simulink model "model_sim_CHBjt9"  (R2023b)
settings: Solver=FixedStepAuto  StartTime=0.0  StopTime=5  FixedStep=1e-6  RelTol=1e-3
InitFcn:
  | sysinit
values from neighbouring files (symbols this model uses):
  C = 0.0234    [sysinit.m]
  f_m = frequency_modulate_start : frequency_modulate_interval : frequency_modulate_end    [simout_chbjt_par.m]    (also in simresjt7.mat = [250 300 350 400 450 500 550 600 650 700 750 800 ... (16 ele)
  L = 0.002    [sysinit.m]
  m = modulate_radio_start : modulate_radio_interval : modulate_radio_end    [simout_chb_par.m]
  R = 1.5    [sysinit.m]
  st = 1e-6    (= 1e-06)    [sysinit.m]
undefined symbols (not defined in the file or in its folder): f, magnitude, Td, Ts2, udc
libraries: spsSeriesRLCBranchLib x123, spsDiodeLib x60, spsIGBTLib x48, spsMeanLib x20, spsCurrentMeasurementLib x16, spsThreePhaseVIMeasurementLib x13, spsOnDelayLib x12, spsUniversalBridgeLib x12, spsMultiWindingTransformerLib x9, spsVoltageMeasurementLib x6, simulink x5, spsPowerLib x2
(part 1 of 3)
settings Model: Creator=Jhchen  LastModifiedBy=ps
settings DataIOCC: ReturnWorkspaceOutputs=off
settings DebuggingCC: RTPrefix=warning

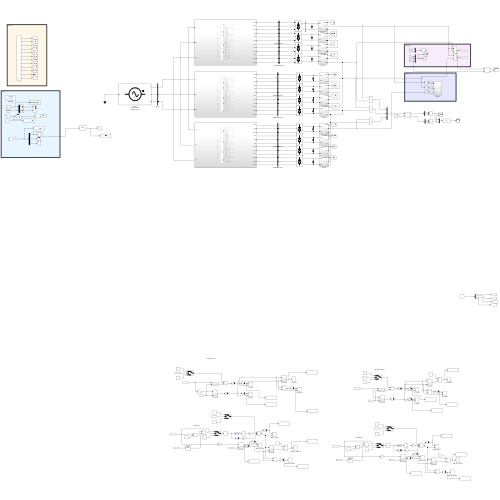
[thumbnail: Simulink's stored preview of the top-level diagram]
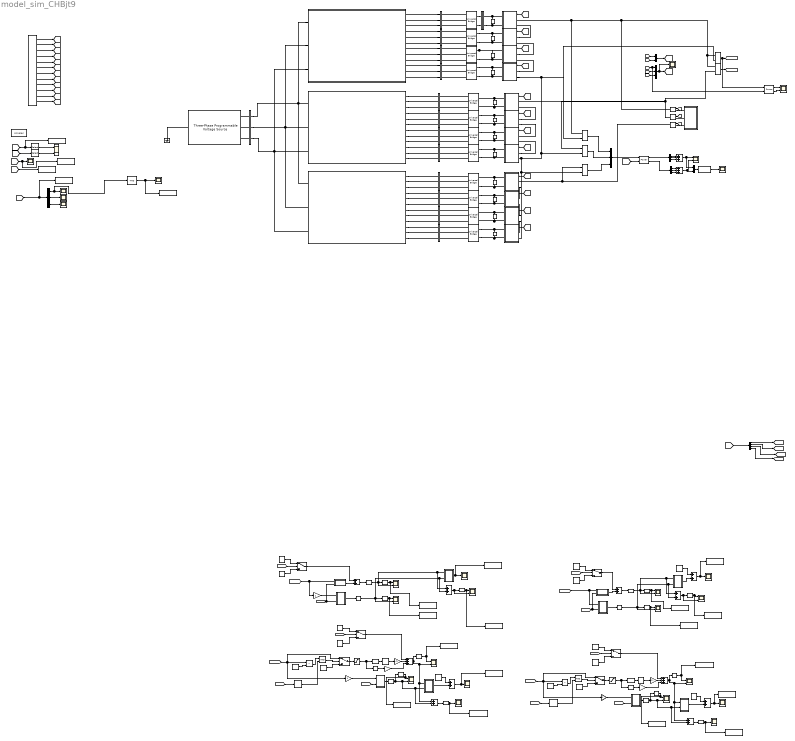
== system model_sim_CHBjt9 ==
  note: PWM_in
  note: result
  note: load_circuit
  note: sampling
  note: 65L4522 6.5KA T2
  note: 34L4520 D1
  note: 34L4520 D2
  note: 65L4522 6KA T1
  3-Phase Programmable Voltage Source7 : spsThreePhaseProgrammableVoltageSourceLib/Three-Phase Programmable Voltage Source  PositiveSequence=[10000 0 50]  VariationEntity=None  VariationType=Step  VariationTypeAlt=Step  VariationStep=0.5  VariationRate=10  VariationMagnitude=0.3  VariationFrequency=2  VariationTiming=[0.05 1]  VariationPhaseA=off  Amplitudes=[1 0.8 1.2 1.0]  TimeValues=[0 0.1 0.15 0.2]  HarmonicGeneration=off  HarmonicA=[5 0.08 -45 2]  HarmonicB=[2 0 0 2]  Timing="[0.1  1]"  BusType=swing  Pref=0  Qref=0  Qmin=-inf  Qmax=inf
  9 : Subsystem  mask{m=m, f=f, f_car=f_m, tt=1/8, ttd=Td}
      mask prompts: m "m_p"; f "f_module"; f_car "f_carrier"; tt "ts"; ttd "td"
      mask DialogControl ParameterGroupVar Prompt: 参数
  ABB_D1_SW1 : Scope  NumInputPorts=2
  ABB_D1_SW2 : Scope  NumInputPorts=2
  ABB_D1_avg1 : Scope  NumInputPorts=2
  ABB_D1_avg2 : Scope  NumInputPorts=2
  ABB_D1_temper{1..3,6} (4 alike) : Scope
  Add{1,4..5,13..14,18..20,30} (9 alike) : Sum
  Add{2..3,6,34} (4 alike) : Sum  Inputs=+++
  Bitwise Operator1 : simulink/Logic and Bit Operations/Bitwise Operator  logicop=NOT  UseBitMask=off  BitMask=bin2dec('11011001')  BitMaskRealWorld=Stored Integer
  Bitwise Operator4 : simulink/Logic and Bit Operations/Bitwise Operator  logicop=NOT  UseBitMask=off  BitMask=bin2dec('11011001')  BitMaskRealWorld=Stored Integer
  C{13..24} (12 alike) : spsSeriesRLCBranchLib/Series RLC Branch  LConnTagsString=__new0  RConnTagsString=__new0  BranchType=C  Resistance=0.0001  Inductance=1.0  SetiL0=off  InitialCurrent=0  Capacitance=C  Setx0=on  InitialVoltage=2500  Measurements=None
  Constant1 : Constant  Value=375
  Constant17 : Constant  Value=125
  Constant{3..8,18,27..29,31} (11 alike) : Constant  Value=0
  Constant2 : Constant  Value=375
  Constant30 : Constant  Value=125
  Current Measurement3 : spsCurrentMeasurementLib/Current Measurement  PhasorSimulation=off  OutputType=Complex  PSBequivalent=0
  Current Measurement4 : spsCurrentMeasurementLib/Current Measurement  PhasorSimulation=off  OutputType=Complex  PSBequivalent=0
  Current Measurement5 : spsCurrentMeasurementLib/Current Measurement  PhasorSimulation=off  OutputType=Complex  PSBequivalent=0
  Demux : Demux  Outputs=3
  Demux1 : Demux  Outputs=3
  Demux2 : Demux  Outputs=3
  Demux3 : Demux
  Fcn : Fcn  Expr=u(1)/sqrt((u(1))^2+(u(2))^2)
  Gain1 : Gain  Gain=0.48e-3
  Gain2 : Gain  Gain=1.46
  Gain26 : Gain
  Gain3 : Gain
  Gain33 : Gain  Gain=0.48e-3
  Gain34 : Gain  Gain=1.46
  Gain35 : Gain
  Ground2 : spsGroundLib/Ground  LConnTagsString=a
  IGCT13 : Subsystem
      settings: PortSchema="{\"entries\":[{\"content\":{\"sides\":[{\"content\":{\"connectorIds\":[\"LConn1\",\"LConn2\"]},\"type\":\"ConnectorPlacement.EquallySpacedRectSide\",\"uuid\":\"3b5227fd-32cc-4097-9a6a-2909540651e9\"},{\"content\":{\"connectorIds\":[\"In1\",\"RConn1\",\"RConn2\"],\"side\":\"RIGHT\"},\"type\":\"ConnectorPlacement.EquallySpacedRectSide\",\"uuid\":\"b0068562-9d9a-456b-acd2-db870c5bcace\"},{\"content\":{\"side\":\"TOP\"},\"type\":\"ConnectorPlacement.EquallySpacedRectSide\",\"uuid\":\"bbecbe08-a8e7-4703-9f6f-443f87d924da\"}]},\"type\":\"ConnectorPlacement.EquallySpacedConnector\",\"uuid\":\"6ec83c7b-e3bb-4502-bc8f-4da9ff103a20\"}],\"packageUris\":[\"http://schema.mathworks.com/mf0/Connector/R2020b\"],\"version\":\"1.0\"}"
  IGCT14 : Subsystem
      settings: PortSchema="{\"entries\":[{\"content\":{\"sides\":[{\"content\":{\"connectorIds\":[\"LConn1\",\"LConn2\"]},\"type\":\"ConnectorPlacement.EquallySpacedRectSide\",\"uuid\":\"3b5227fd-32cc-4097-9a6a-2909540651e9\"},{\"content\":{\"connectorIds\":[\"In1\",\"RConn1\",\"RConn2\"],\"side\":\"RIGHT\"},\"type\":\"ConnectorPlacement.EquallySpacedRectSide\",\"uuid\":\"b0068562-9d9a-456b-acd2-db870c5bcace\"},{\"content\":{\"side\":\"TOP\"},\"type\":\"ConnectorPlacement.EquallySpacedRectSide\",\"uuid\":\"bbecbe08-a8e7-4703-9f6f-443f87d924da\"}]},\"type\":\"ConnectorPlacement.EquallySpacedConnector\",\"uuid\":\"6ec83c7b-e3bb-4502-bc8f-4da9ff103a20\"}],\"packageUris\":[\"http://schema.mathworks.com/mf0/Connector/R2020b\"],\"version\":\"1.0\"}"
  IGCT15 : Subsystem
      settings: PortSchema="{\"entries\":[{\"content\":{\"sides\":[{\"content\":{\"connectorIds\":[\"LConn1\",\"LConn2\"]},\"type\":\"ConnectorPlacement.EquallySpacedRectSide\",\"uuid\":\"3b5227fd-32cc-4097-9a6a-2909540651e9\"},{\"content\":{\"connectorIds\":[\"In1\",\"RConn1\",\"RConn2\"],\"side\":\"RIGHT\"},\"type\":\"ConnectorPlacement.EquallySpacedRectSide\",\"uuid\":\"b0068562-9d9a-456b-acd2-db870c5bcace\"},{\"content\":{\"side\":\"TOP\"},\"type\":\"ConnectorPlacement.EquallySpacedRectSide\",\"uuid\":\"bbecbe08-a8e7-4703-9f6f-443f87d924da\"}]},\"type\":\"ConnectorPlacement.EquallySpacedConnector\",\"uuid\":\"6ec83c7b-e3bb-4502-bc8f-4da9ff103a20\"}],\"packageUris\":[\"http://schema.mathworks.com/mf0/Connector/R2020b\"],\"version\":\"1.0\"}"
  IGCT16 : Subsystem
      settings: PortSchema="{\"entries\":[{\"content\":{\"sides\":[{\"content\":{\"connectorIds\":[\"LConn1\",\"LConn2\"]},\"type\":\"ConnectorPlacement.EquallySpacedRectSide\",\"uuid\":\"3b5227fd-32cc-4097-9a6a-2909540651e9\"},{\"content\":{\"connectorIds\":[\"In1\",\"RConn1\",\"RConn2\"],\"side\":\"RIGHT\"},\"type\":\"ConnectorPlacement.EquallySpacedRectSide\",\"uuid\":\"b0068562-9d9a-456b-acd2-db870c5bcace\"},{\"content\":{\"side\":\"TOP\"},\"type\":\"ConnectorPlacement.EquallySpacedRectSide\",\"uuid\":\"bbecbe08-a8e7-4703-9f6f-443f87d924da\"}]},\"type\":\"ConnectorPlacement.EquallySpacedConnector\",\"uuid\":\"6ec83c7b-e3bb-4502-bc8f-4da9ff103a20\"}],\"packageUris\":[\"http://schema.mathworks.com/mf0/Connector/R2020b\"],\"version\":\"1.0\"}"
  IGCT17 : Subsystem
      settings: PortSchema="{\"entries\":[{\"content\":{\"sides\":[{\"content\":{\"connectorIds\":[\"LConn1\",\"LConn2\"]},\"type\":\"ConnectorPlacement.EquallySpacedRectSide\",\"uuid\":\"3b5227fd-32cc-4097-9a6a-2909540651e9\"},{\"content\":{\"connectorIds\":[\"In1\",\"RConn1\",\"RConn2\"],\"side\":\"RIGHT\"},\"type\":\"ConnectorPlacement.EquallySpacedRectSide\",\"uuid\":\"b0068562-9d9a-456b-acd2-db870c5bcace\"},{\"content\":{\"side\":\"TOP\"},\"type\":\"ConnectorPlacement.EquallySpacedRectSide\",\"uuid\":\"bbecbe08-a8e7-4703-9f6f-443f87d924da\"}]},\"type\":\"ConnectorPlacement.EquallySpacedConnector\",\"uuid\":\"6ec83c7b-e3bb-4502-bc8f-4da9ff103a20\"}],\"packageUris\":[\"http://schema.mathworks.com/mf0/Connector/R2020b\"],\"version\":\"1.0\"}"
  IGCT18 : Subsystem
      settings: PortSchema="{\"entries\":[{\"content\":{\"sides\":[{\"content\":{\"connectorIds\":[\"LConn1\",\"LConn2\"]},\"type\":\"ConnectorPlacement.EquallySpacedRectSide\",\"uuid\":\"3b5227fd-32cc-4097-9a6a-2909540651e9\"},{\"content\":{\"connectorIds\":[\"In1\",\"RConn1\",\"RConn2\"],\"side\":\"RIGHT\"},\"type\":\"ConnectorPlacement.EquallySpacedRectSide\",\"uuid\":\"b0068562-9d9a-456b-acd2-db870c5bcace\"},{\"content\":{\"side\":\"TOP\"},\"type\":\"ConnectorPlacement.EquallySpacedRectSide\",\"uuid\":\"bbecbe08-a8e7-4703-9f6f-443f87d924da\"}]},\"type\":\"ConnectorPlacement.EquallySpacedConnector\",\"uuid\":\"6ec83c7b-e3bb-4502-bc8f-4da9ff103a20\"}],\"packageUris\":[\"http://schema.mathworks.com/mf0/Connector/R2020b\"],\"version\":\"1.0\"}"
  IGCT19 : Subsystem
      settings: PortSchema="{\"entries\":[{\"content\":{\"sides\":[{\"content\":{\"connectorIds\":[\"LConn1\",\"LConn2\"]},\"type\":\"ConnectorPlacement.EquallySpacedRectSide\",\"uuid\":\"3b5227fd-32cc-4097-9a6a-2909540651e9\"},{\"content\":{\"connectorIds\":[\"In1\",\"RConn1\",\"RConn2\"],\"side\":\"RIGHT\"},\"type\":\"ConnectorPlacement.EquallySpacedRectSide\",\"uuid\":\"b0068562-9d9a-456b-acd2-db870c5bcace\"},{\"content\":{\"side\":\"TOP\"},\"type\":\"ConnectorPlacement.EquallySpacedRectSide\",\"uuid\":\"bbecbe08-a8e7-4703-9f6f-443f87d924da\"}]},\"type\":\"ConnectorPlacement.EquallySpacedConnector\",\"uuid\":\"6ec83c7b-e3bb-4502-bc8f-4da9ff103a20\"}],\"packageUris\":[\"http://schema.mathworks.com/mf0/Connector/R2020b\"],\"version\":\"1.0\"}"
  IGCT20 : Subsystem
      settings: PortSchema="{\"entries\":[{\"content\":{\"sides\":[{\"content\":{\"connectorIds\":[\"LConn1\",\"LConn2\"]},\"type\":\"ConnectorPlacement.EquallySpacedRectSide\",\"uuid\":\"3b5227fd-32cc-4097-9a6a-2909540651e9\"},{\"content\":{\"connectorIds\":[\"In1\",\"RConn1\",\"RConn2\"],\"side\":\"RIGHT\"},\"type\":\"ConnectorPlacement.EquallySpacedRectSide\",\"uuid\":\"b0068562-9d9a-456b-acd2-db870c5bcace\"},{\"content\":{\"side\":\"TOP\"},\"type\":\"ConnectorPlacement.EquallySpacedRectSide\",\"uuid\":\"bbecbe08-a8e7-4703-9f6f-443f87d924da\"}]},\"type\":\"ConnectorPlacement.EquallySpacedConnector\",\"uuid\":\"6ec83c7b-e3bb-4502-bc8f-4da9ff103a20\"}],\"packageUris\":[\"http://schema.mathworks.com/mf0/Connector/R2020b\"],\"version\":\"1.0\"}"
  IGCT21 : Subsystem
      settings: PortSchema="{\"entries\":[{\"content\":{\"sides\":[{\"content\":{\"connectorIds\":[\"LConn1\",\"LConn2\"]},\"type\":\"ConnectorPlacement.EquallySpacedRectSide\",\"uuid\":\"3b5227fd-32cc-4097-9a6a-2909540651e9\"},{\"content\":{\"connectorIds\":[\"In1\",\"RConn1\",\"RConn2\"],\"side\":\"RIGHT\"},\"type\":\"ConnectorPlacement.EquallySpacedRectSide\",\"uuid\":\"b0068562-9d9a-456b-acd2-db870c5bcace\"},{\"content\":{\"side\":\"TOP\"},\"type\":\"ConnectorPlacement.EquallySpacedRectSide\",\"uuid\":\"bbecbe08-a8e7-4703-9f6f-443f87d924da\"}]},\"type\":\"ConnectorPlacement.EquallySpacedConnector\",\"uuid\":\"6ec83c7b-e3bb-4502-bc8f-4da9ff103a20\"}],\"packageUris\":[\"http://schema.mathworks.com/mf0/Connector/R2020b\"],\"version\":\"1.0\"}"
  IGCT22 : Subsystem
      settings: PortSchema="{\"entries\":[{\"content\":{\"sides\":[{\"content\":{\"connectorIds\":[\"LConn1\",\"LConn2\"]},\"type\":\"ConnectorPlacement.EquallySpacedRectSide\",\"uuid\":\"3b5227fd-32cc-4097-9a6a-2909540651e9\"},{\"content\":{\"connectorIds\":[\"In1\",\"RConn1\",\"RConn2\"],\"side\":\"RIGHT\"},\"type\":\"ConnectorPlacement.EquallySpacedRectSide\",\"uuid\":\"b0068562-9d9a-456b-acd2-db870c5bcace\"},{\"content\":{\"side\":\"TOP\"},\"type\":\"ConnectorPlacement.EquallySpacedRectSide\",\"uuid\":\"bbecbe08-a8e7-4703-9f6f-443f87d924da\"}]},\"type\":\"ConnectorPlacement.EquallySpacedConnector\",\"uuid\":\"6ec83c7b-e3bb-4502-bc8f-4da9ff103a20\"}],\"packageUris\":[\"http://schema.mathworks.com/mf0/Connector/R2020b\"],\"version\":\"1.0\"}"
  IGCT23 : Subsystem
      settings: PortSchema="{\"entries\":[{\"content\":{\"sides\":[{\"content\":{\"connectorIds\":[\"LConn1\",\"LConn2\"]},\"type\":\"ConnectorPlacement.EquallySpacedRectSide\",\"uuid\":\"3b5227fd-32cc-4097-9a6a-2909540651e9\"},{\"content\":{\"connectorIds\":[\"In1\",\"RConn1\",\"RConn2\"],\"side\":\"RIGHT\"},\"type\":\"ConnectorPlacement.EquallySpacedRectSide\",\"uuid\":\"b0068562-9d9a-456b-acd2-db870c5bcace\"},{\"content\":{\"side\":\"TOP\"},\"type\":\"ConnectorPlacement.EquallySpacedRectSide\",\"uuid\":\"bbecbe08-a8e7-4703-9f6f-443f87d924da\"}]},\"type\":\"ConnectorPlacement.EquallySpacedConnector\",\"uuid\":\"6ec83c7b-e3bb-4502-bc8f-4da9ff103a20\"}],\"packageUris\":[\"http://schema.mathworks.com/mf0/Connector/R2020b\"],\"version\":\"1.0\"}"
  IGCT24 : Subsystem
      settings: PortSchema="{\"entries\":[{\"content\":{\"sides\":[{\"content\":{\"connectorIds\":[\"LConn1\",\"LConn2\"]},\"type\":\"ConnectorPlacement.EquallySpacedRectSide\",\"uuid\":\"3b5227fd-32cc-4097-9a6a-2909540651e9\"},{\"content\":{\"connectorIds\":[\"In1\",\"RConn1\",\"RConn2\"],\"side\":\"RIGHT\"},\"type\":\"ConnectorPlacement.EquallySpacedRectSide\",\"uuid\":\"b0068562-9d9a-456b-acd2-db870c5bcace\"},{\"content\":{\"side\":\"TOP\"},\"type\":\"ConnectorPlacement.EquallySpacedRectSide\",\"uuid\":\"bbecbe08-a8e7-4703-9f6f-443f87d924da\"}]},\"type\":\"ConnectorPlacement.EquallySpacedConnector\",\"uuid\":\"6ec83c7b-e3bb-4502-bc8f-4da9ff103a20\"}],\"packageUris\":[\"http://schema.mathworks.com/mf0/Connector/R2020b\"],\"version\":\"1.0\"}"
  LOAD1 : Subsystem
  Logical Operator : Logic  AllPortsSameDT=off  OutDataTypeStr=boolean
  Logical Operator1 : Logic  AllPortsSameDT=off  OutDataTypeStr=boolean
  Math Function1 : Math  Operator=magnitude^2  SignedPower=on
  Math Function11 : Math  Operator=magnitude^2  SignedPower=on
  Mean{1,4,12..13,25,27,39,83} (8 alike) : spsMeanLib/Mean  Freq=2000  Vinit=0  Ts=1e-6
  Mean{15..16,26,28} (4 alike) : spsMeanLib/Mean  Freq=f  Vinit=0  Ts=Ts2
  Mean{2..3,5,17,24,58,82,84} (8 alike) : spsMeanLib/Mean  Freq=f  Vinit=0  Ts=1e-6
  Mux2 : Mux  Inputs=3
  Mux3 : Mux  Inputs=2
  Mux4 : Mux  Inputs=3
  Mux5 : Mux  Inputs=2
  Power : spsPowerLib/Power  Freq=50  Vinit=[1, 0]  Iinit=[1, 0]  Ts=0
  Power1 : spsPowerLib/Power  Freq=50  Vinit=[1, 0]  Iinit=[1, 0]  Ts=0
  RMS1 : spsRMSLib/RMS  TrueRMS=on  Freq=2000  RMSInit=0  Ts=1e-6
  RMS23 : spsRMSLib/RMS  TrueRMS=on  Freq=2000  RMSInit=0  Ts=1e-6
  Relational Operator : RelationalOperator  Operator=>  OutDataTypeStr=boolean  RndMeth=Simplest  InputSameDT=off
  Relational Operator1 : RelationalOperator  Operator=>  OutDataTypeStr=boolean  RndMeth=Simplest  InputSameDT=off
  Saturation1 : Saturate  UpperLimit=5500  LowerLimit=0
  Saturation11 : Saturate  UpperLimit=5500  LowerLimit=0
  Scope : Scope  NumInputPorts=2
  Scope{2..6,10,13} (7 alike) : Scope
  Scope11 : Scope  NumInputPorts=2
  Scope12 : Scope  NumInputPorts=2
  Selector : Selector  InputPortWidth=2  IndexOptions=Index vector (dialog)  Indices=[1]  OutputSizes=1
  Selector1 : Selector  InputPortWidth=3  IndexOptions=Index vector (dialog)  Indices=[1]  OutputSizes=1
  Subsystem1 : Subsystem
  Subsystem14 : Subsystem
  Subsystem15 : Subsystem
  Subsystem16 : Subsystem
  Subsystem17 : Subsystem
  Subsystem18 : Subsystem
  Subsystem2 : Subsystem
  Subsystem3 : Subsystem
  Subsystem4 : Subsystem
  Subsystem48 : Subsystem
  Subsystem49 : Subsystem
  Subsystem5 : Subsystem
  Subsystem6 : Subsystem
  Subsystem9 : Subsystem
  Switch{,1..3,6,9} (6 alike) : Switch  Criteria=u2 > Threshold  SaturateOnIntegerOverflow=off  InputSameDT=off
  T1_SW2 : Scope  NumInputPorts=2
  T1_SW3 : Scope  NumInputPorts=2
  T1_avg2 : Scope  NumInputPorts=2
  T1_avg3 : Scope  NumInputPorts=2
  THD : spsTHDLib/THD  Freq=50  Ts=0
  To Workspace : ToWorkspace  VariableName=current_grid  SaveFormat=Structure With Time  SampleTime=-1
  To Workspace1 : ToWorkspace  VariableName=current_load  SaveFormat=Structure With Time  SampleTime=-1
  To Workspace10 : ToWorkspace  VariableName=D1_sw  SaveFormat=Structure With Time  SampleTime=-1
  To Workspace11 : ToWorkspace  VariableName=D1_all  SaveFormat=Structure With Time  SampleTime=-1
  To Workspace12 : ToWorkspace  VariableName=T2_tem  SaveFormat=Structure With Time  SampleTime=-1
  To Workspace13 : ToWorkspace  VariableName=T2_all  SaveFormat=Structure With Time  SampleTime=-1
  To Workspace14 : ToWorkspace  VariableName=T2_onavg  SaveFormat=Structure With Time  SampleTime=-1
  To Workspace15 : ToWorkspace  VariableName=T2_sw  SaveFormat=Structure With Time  SampleTime=-1
  To Workspace16 : ToWorkspace  VariableName=D2_sw  SaveFormat=Structure With Time  SampleTime=-1
  To Workspace17 : ToWorkspace  VariableName=D2_all  SaveFormat=Structure With Time  SampleTime=-1
  To Workspace18 : ToWorkspace  VariableName=D2_onavg  SaveFormat=Structure With Time  SampleTime=-1
  To Workspace19 : ToWorkspace  VariableName=D1_tem  SaveFormat=Structure With Time  SampleTime=-1
  To Workspace2 : ToWorkspace  VariableName=voltage_load  SaveFormat=Structure With Time  SampleTime=-1
  To Workspace20 : ToWorkspace  VariableName=D2_tem  SaveFormat=Structure With Time  SampleTime=-1
  To Workspace3 : ToWorkspace  VariableName=voltage_dc  SaveFormat=Structure With Time  SampleTime=-1
  To Workspace4 : ToWorkspace  VariableName=T1_onavg  SaveFormat=Structure With Time  SampleTime=-1
  To Workspace5 : ToWorkspace  VariableName=THD  SaveFormat=Structure With Time  SampleTime=-1
  To Workspace6 : ToWorkspace  VariableName=T1_sw  SaveFormat=Structure With Time  SampleTime=-1
  To Workspace7 : ToWorkspace  VariableName=T1_tem  SaveFormat=Structure With Time  SampleTime=-1
  To Workspace8 : ToWorkspace  VariableName=T1_all  SaveFormat=Structure With Time  SampleTime=-1
  To Workspace9 : ToWorkspace  VariableName=D1_onavg  SaveFormat=Structure With Time  SampleTime=-1
  Universal Bridge{13..24} (12 alike) : spsUniversalBridgeLib/Universal Bridge  Arms=3  SnubberResistance=1e5  SnubberCapacitance=inf  Device=Diodes  Ron=1e-3  Lon=0  ForwardVoltages="[  0  0  ]"  ForwardVoltage=0  GTOparameters=[ 10e-6 , 20e-6 ]  IGBTparameters=[ 1e-6 , 2e-6 ]  Measurements=None  Measurements_2=None  converterType=Rectifier
  Voltage Measurement{3..7} (5 alike) : spsVoltageMeasurementLib/Voltage Measurement  PhasorSimulation=off  OutputType=Complex  PSBequivalent=0
  grid1 : spsThreePhaseVIMeasurementLib/Three-Phase V-I Measurement  VoltageMeasurement=phase-to-ground  SetLabelV=on  LabelV=Vgrid1  Vpu=off  VpuLL=off  CurrentMeasurement=yes  SetLabelI=on  LabelI=Igrid1  Ipu=off  Pbase=1e3  Vbase=380  OutputType=Magnitude  PhasorSimulation=off  PSBequivalent=0
  powergui : sps_lib/powergui  Priority=1  SimulationMode=Discrete  SampleTime=st  frequency=60  Iterations=50  frequencyindice=50  Pbase=100e6  ErrMax=1e-4  UnitsV=kV  UnitsW=MW  buscounter=0  FunctionMessages=off  echomessages=off  EnableUseOfTLC=off  CurrentSourceSwitches=off  DisableSnubberDevices=off  DisableRonSwitches=off  DisableVfSwitches=off  DisplayEquations=off  AutomaticDiscreteSolvers=off  SolverType=Tustin/Backward Euler (TBE)  Interpol=off  ExternalGateDelay=off  methode=off  Ts=100  x0status=blocks  SPID=on  SwTol=0  HookPort=off  NonlinearTolerance=1e-4  nMaxIteration=100  ContinueOnMaxIteration=off  RestoreLinks=warning  ResistiveCurrentMeasurement=off  Frange=[0:2:500]  Ylog=off  Xlog=on  ShowGrid=off  save=off  variable=ZData  structure=0  ZoomFFT=off  StartTime=0.0  cycles=1  DisplayStyle=1  fundamental=60  FreqAxis=off  MaxFrequency=1000  frequencyindicesteady=1  RmsSteady=1  display=off
  secondary1.13 : spsThreePhaseVIMeasurementLib/Three-Phase V-I Measurement  VoltageMeasurement=phase-to-phase  SetLabelV=on  LabelV=Vsecondary_a1  Vpu=off  VpuLL=off  CurrentMeasurement=yes  SetLabelI=on  LabelI=Isecondary_a1  Ipu=off  Pbase=1e3  Vbase=380  OutputType=Magnitude  PhasorSimulation=off  PSBequivalent=0
  secondary1.14 : spsThreePhaseVIMeasurementLib/Three-Phase V-I Measurement  VoltageMeasurement=phase-to-phase  SetLabelV=on  LabelV=Vsecondary_c2  Vpu=off  VpuLL=off  CurrentMeasurement=yes  SetLabelI=on  LabelI=Isecondary_c2  Ipu=off  Pbase=1e3  Vbase=380  OutputType=Magnitude  PhasorSimulation=off  PSBequivalent=0
  secondary1.15 : spsThreePhaseVIMeasurementLib/Three-Phase V-I Measurement  VoltageMeasurement=phase-to-phase  SetLabelV=on  LabelV=Vsecondary_c3  Vpu=off  VpuLL=off  CurrentMeasurement=yes  SetLabelI=on  LabelI=Isecondary_c3  Ipu=off  Pbase=1e3  Vbase=380  OutputType=Magnitude  PhasorSimulation=off  PSBequivalent=0
  secondary1.16 : spsThreePhaseVIMeasurementLib/Three-Phase V-I Measurement  VoltageMeasurement=phase-to-phase  SetLabelV=on  LabelV=Vsecondary_c4  Vpu=off  VpuLL=off  CurrentMeasurement=yes  SetLabelI=on  LabelI=Isecondary_c4  Ipu=off  Pbase=1e3  Vbase=380  OutputType=Magnitude  PhasorSimulation=off  PSBequivalent=0
  secondary1.17 : spsThreePhaseVIMeasurementLib/Three-Phase V-I Measurement  VoltageMeasurement=phase-to-phase  SetLabelV=on  LabelV=Vsecondary_a2  Vpu=off  VpuLL=off  CurrentMeasurement=yes  SetLabelI=on  LabelI=Isecondary_a2  Ipu=off  Pbase=1e3  Vbase=380  OutputType=Magnitude  PhasorSimulation=off  PSBequivalent=0
  secondary1.18 : spsThreePhaseVIMeasurementLib/Three-Phase V-I Measurement  VoltageMeasurement=phase-to-phase  SetLabelV=on  LabelV=Vsecondary_a3  Vpu=off  VpuLL=off  CurrentMeasurement=yes  SetLabelI=on  LabelI=Isecondary_a3  Ipu=off  Pbase=1e3  Vbase=380  OutputType=Magnitude  PhasorSimulation=off  PSBequivalent=0
  secondary1.19 : spsThreePhaseVIMeasurementLib/Three-Phase V-I Measurement  VoltageMeasurement=phase-to-phase  SetLabelV=on  LabelV=Vsecondary_a4  Vpu=off  VpuLL=off  CurrentMeasurement=yes  SetLabelI=on  LabelI=Isecondary_a4  Ipu=off  Pbase=1e3  Vbase=380  OutputType=Magnitude  PhasorSimulation=off  PSBequivalent=0
  secondary1.20 : spsThreePhaseVIMeasurementLib/Three-Phase V-I Measurement  VoltageMeasurement=phase-to-phase  SetLabelV=on  LabelV=Vsecondary_b1  Vpu=off  VpuLL=off  CurrentMeasurement=yes  SetLabelI=on  LabelI=Isecondary_b1  Ipu=off  Pbase=1e3  Vbase=380  OutputType=Magnitude  PhasorSimulation=off  PSBequivalent=0
  secondary1.21 : spsThreePhaseVIMeasurementLib/Three-Phase V-I Measurement  VoltageMeasurement=phase-to-phase  SetLabelV=on  LabelV=Vsecondary_b2  Vpu=off  VpuLL=off  CurrentMeasurement=yes  SetLabelI=on  LabelI=Isecondary_b2  Ipu=off  Pbase=1e3  Vbase=380  OutputType=Magnitude  PhasorSimulation=off  PSBequivalent=0
  secondary1.22 : spsThreePhaseVIMeasurementLib/Three-Phase V-I Measurement  VoltageMeasurement=phase-to-phase  SetLabelV=on  LabelV=Vsecondary_b3  Vpu=off  VpuLL=off  CurrentMeasurement=yes  SetLabelI=on  LabelI=Isecondary_b3  Ipu=off  Pbase=1e3  Vbase=380  OutputType=Magnitude  PhasorSimulation=off  PSBequivalent=0
  secondary1.23 : spsThreePhaseVIMeasurementLib/Three-Phase V-I Measurement  VoltageMeasurement=phase-to-phase  SetLabelV=on  LabelV=Vsecondary_b4  Vpu=off  VpuLL=off  CurrentMeasurement=yes  SetLabelI=on  LabelI=Isecondary_b4  Ipu=off  Pbase=1e3  Vbase=380  OutputType=Magnitude  PhasorSimulation=off  PSBequivalent=0
  secondary1.24 : spsThreePhaseVIMeasurementLib/Three-Phase V-I Measurement  VoltageMeasurement=phase-to-phase  SetLabelV=on  LabelV=Vsecondary_c1  Vpu=off  VpuLL=off  CurrentMeasurement=yes  SetLabelI=on  LabelI=Isecondary_c1  Ipu=off  Pbase=1e3  Vbase=380  OutputType=Magnitude  PhasorSimulation=off  PSBequivalent=0
  t1_temper5 : Scope
  t1_temper7 : Scope  NumInputPorts=2
  t1_temper8 : Scope  NumInputPorts=2
  t1_temper9 : Scope
  tag scope: IloadA=global, IloadB=global, IloadC=global, VloadABline=global, VloadAphase=global, pwm10=global, pwm11=global, pwm12=global, pwm1=global, pwm2=global, pwm3=global, pwm4=global, pwm5=global, pwm6=global, pwm7=global, pwm8=global, pwm9=global
  wires:
  [Vload] -> To Workspace2/1, Selector/1
  Selector/1 -> Scope/1
  [Iload] -> Selector1/1
  Selector1/1 -> Scope/2
  [IloadA] -> To Workspace1/1
  [Udc] -> To Workspace3/1, Scope3/1
  9/1(Output) -> [pwm1]
  9/2(Output1) -> [pwm2]
  9/3(Output2) -> [pwm3]
  9/4(Output3) -> [pwm4]
  9/5(Output4) -> [pwm5]
  9/6(Output5) -> [pwm6]
  9/7(Output6) -> [pwm7]
  9/8(Output7) -> [pwm8]
  9/9(Output8) -> [pwm9]
  9/10(Output9) -> [pwm10]
  9/11(Output10) -> [pwm11]
  9/12(Output11) -> [pwm12]
  [Igrid1] -> Demux/1, To Workspace/1
  Demux/1 -> THD/1, Scope4/1
  Demux/2 -> Scope5/1
  Demux/3 -> Scope6/1
  [pwm7] -> IGCT22/1(PWM)
  [pwm8] -> IGCT23/1(PWM)
  [pwm9] -> IGCT24/1(PWM)
  [pwm10] -> IGCT14/1(PWM)
  [pwm11] -> IGCT15/1(PWM)
  [pwm12] -> IGCT16/1(PWM)
  [pwm6] -> IGCT21/1(PWM)
  [pwm5] -> IGCT20/1(PWM)
  [pwm4] -> IGCT19/1(PWM)
  [pwm3] -> IGCT18/1(PWM)
  [pwm2] -> IGCT17/1(PWM)
  [pwm1] -> IGCT13/1(PWM)
  Mux3/1 -> [Vload]
  [VloadAphase] -> Mux3/1
  Current Measurement3/1 -> [IloadA]
  [IloadB] -> Mux2/2
  Voltage Measurement3/1 -> [VloadABline]
  Mux2/1 -> Scope10/1, [Iload]
  Current Measurement4/1 -> [IloadB]
  Current Measurement5/1 -> [IloadC]
  [IloadC] -> Mux2/3
  [IloadA] -> Power/2, Mux2/1
  [VloadABline] -> Mux3/2
  Voltage Measurement4/1 -> Power/1, [VloadAphase]
  Power/1 -> Scope11/1
  Power/2 -> Scope11/2
  Voltage Measurement7/1 -> Mux4/1
  Voltage Measurement5/1 -> Mux4/2
  Voltage Measurement6/1 -> Mux4/3
  Mux4/1 -> Power1/1
  [Iload] -> Power1/2
  Power1/2 -> Demux1/1
  Power1/1 -> Demux2/1
  Demux2/1 -> Add2/1
  Demux2/2 -> Add2/2
  Demux2/3 -> Add2/3
  Demux1/2 -> Add3/2
  Demux1/3 -> Add3/3
  Demux1/1 -> Add3/1
  Add2/1 -> Mux5/1, Scope12/1
  Add3/1 -> Mux5/2, Scope12/2
  Mux5/1 -> Fcn/1
  Fcn/1 -> Scope13/1
  THD/1 -> To Workspace5/1, Scope2/1
  [IloadA] -> Switch/1, Gain35/1, Relational Operator/1
  Mean17/1 -> To Workspace8/1, t1_temper7/1
  Add13/1 -> t1_temper7/2, Mean17/1
  Demux3/1 -> [T1]
  Gain34/1 -> Add34/3
  Constant28/1 -> Switch/3
  Bitwise Operator4/1 -> Logical Operator/2
  Constant17/1 -> Switch6/3
  Constant2/1 -> Switch2/3
  Demux3/2 -> [T2]
  Mean16/1 -> To Workspace6/1, T1_SW2/1
  [T1] -> Switch2/2
  Add34/1 -> Add30/1, Subsystem49/1(In1), ABB_D1_avg2/2, Mean82/1
  Add20/1 -> Mean27/1
  Add19/1 -> t1_temper8/2, Mean24/1
  Gain26/1 -> Subsystem9/1(In1)
  Switch6/1 -> Add14/1
  Mean12/1 -> Subsystem18/2(In2), Add13/2, T1_SW2/2, Mean16/1
  Subsystem17/1(Out1) -> Add14/2
  Add30/1 -> Mean58/1
  Constant6/1 -> Add4/1
  Mean58/1 -> ABB_D1_temper6/1, To Workspace11/1
  Mean28/1 -> To Workspace15/1, T1_SW3/1
  [T1] -> Subsystem9/2(In2), Subsystem17/2(In2)
  [IloadA] -> Gain26/1, Subsystem17/1(In1)
  Add5/1 -> Mean2/1
  [IloadA] -> Subsystem16/1(In1), Subsystem14/1(In1)
  Mean5/1 -> ABB_D1_SW1/1, To Workspace16/1
  RMS1/1 -> Math Function1/1
  Add4/1 -> To Workspace19/1, ABB_D1_temper2/1
  Add6/1 -> Mean3/1, ABB_D1_avg1/2, Subsystem6/1(In1), Add5/1
  Relational Operator1/1 -> Logical Operator1/1
  [T2] -> Switch3/2
  Constant7/1 -> Switch3/1
  Gain1/1 -> Add6/2
  [IloadA] -> Relational Operator1/1, Gain3/1, Switch1/1
  Subsystem9/1(Out1) -> Mean12/1
  Add1/1 -> To Workspace20/1, ABB_D1_temper1/1
  Gain3/1 -> Subsystem5/1(In1)
  Mean3/1 -> To Workspace18/1, ABB_D1_avg1/1
  Demux3/3 -> [T3]
  Logical Operator1/1 -> Switch1/2
  Switch1/1 -> Saturation1/1
  Mean4/1 -> ABB_D1_SW1/2, Subsystem6/2(In2), Add5/2, Mean5/1
  Saturation1/1 -> RMS1/1, Mean1/1
  Add18/1 -> To Workspace12/1, t1_temper9/1
  Constant18/1 -> Switch6/1
  Subsystem16/1(Out1) -> Mean25/1
  Constant29/1 -> Add18/1
  [T2] -> Subsystem14/2(In2), Subsystem16/2(In2)
  Subsystem15/1(Out1) -> Add18/2
  Mean27/1 -> T1_avg3/2, Mean26/1, Subsystem15/1(In1), Add19/1
  Relational Operator/1 -> Logical Operator/1
  Subsystem14/1(Out1) -> Add20/2
  [T1] -> Switch6/2
  Constant31/1 -> Switch9/1
  Constant1/1 -> Switch3/3
  Mean24/1 -> To Workspace13/1, t1_temper8/1
  RMS23/1 -> Math Function11/1
  [T2] -> Switch9/2
  Mean84/1 -> To Workspace10/1, ABB_D1_SW2/1
  Saturation11/1 -> Mean39/1, RMS23/1
  Switch9/1 -> Add20/1
  Constant30/1 -> Switch9/3
  Constant5/1 -> Switch1/3
  Mean25/1 -> Subsystem15/2(In2), Add19/2, T1_SW3/2, Mean28/1
  Mean82/1 -> ABB_D1_avg2/1, To Workspace9/1
  Gain35/1 -> Subsystem48/1(In1)
  Math Function11/1 -> Gain33/1
  Bitwise Operator1/1 -> Logical Operator1/2
  Add14/1 -> Mean13/1
  Mean26/1 -> To Workspace14/1, T1_avg3/1
  Mean39/1 -> Gain34/1
  Switch2/1 -> Add34/1
  Constant27/1 -> Relational Operator/2
  Subsystem48/1(Out1) -> Mean83/1
  Subsystem18/1(Out1) -> To Workspace7/1, t1_temper5/1
  Mean15/1 -> To Workspace4/1, T1_avg2/1
  [T3] -> Subsystem48/2(In2)
  Demux3/4 -> [T4]
  Constant8/1 -> Add1/1
  Gain2/1 -> Add6/3
  Mean13/1 -> T1_avg2/2, Mean15/1, Subsystem18/1(In1), Add13/1
  [T3] -> Bitwise Operator4/1
  [T4] -> Subsystem5/2(In2)
  Subsystem6/1(Out1) -> Add1/2
  Math Function1/1 -> Gain1/1
  Mean2/1 -> To Workspace17/1, ABB_D1_temper3/1
  Subsystem49/1(Out1) -> Add4/2
  [T4] -> Bitwise Operator1/1
  Logical Operator/1 -> Switch/2
  Constant3/1 -> Switch2/1
  Switch/1 -> Saturation11/1
  Constant4/1 -> Relational Operator1/2
  Mean1/1 -> Gain2/1
  [pwm1] -> Demux3/1
  Mean83/1 -> Mean84/1, Add30/2, Subsystem49/2(In2), ABB_D1_SW2/2
  Switch3/1 -> Add6/1
  Subsystem5/1(Out1) -> Mean4/1
  Gain33/1 -> Add34/2
  connections:
  3-Phase Programmable Voltage Source7/LConn1 -- Ground2/LConn1
  Subsystem3/RConn8 -- secondary1.15/LConn2
  Universal Bridge21/LConn1 -- secondary1.23/RConn1
  Universal Bridge14/LConn2 -- secondary1.16/RConn2
  Universal Bridge15/LConn2 -- secondary1.15/RConn2
  Subsystem2/RConn11 -- secondary1.23/LConn2
  Universal Bridge16/LConn2 -- secondary1.22/RConn2
  Subsystem3/RConn9 -- secondary1.15/LConn3
  Subsystem2/RConn12 -- secondary1.23/LConn3
  Universal Bridge24/LConn1 -- secondary1.24/RConn1
  Universal Bridge16/LConn1 -- secondary1.22/RConn1
  Subsystem2/RConn9 -- secondary1.22/LConn3
  Subsystem2/RConn8 -- secondary1.22/LConn2
  Universal Bridge21/LConn2 -- secondary1.23/RConn2
  Universal Bridge16/LConn3 -- secondary1.22/RConn3
  Universal Bridge22/LConn1 -- secondary1.14/RConn1
  Subsystem2/RConn7 -- secondary1.22/LConn1
  Universal Bridge15/LConn1 -- secondary1.15/RConn1
  Universal Bridge22/LConn2 -- secondary1.14/RConn2
  Subsystem3/RConn2 -- secondary1.24/LConn2
  Subsystem3/RConn6 -- secondary1.14/LConn3
  Universal Bridge24/LConn2 -- secondary1.24/RConn2
  Subsystem3/RConn11 -- secondary1.16/LConn2
  Subsystem3/RConn7 -- secondary1.15/LConn1
  Subsystem3/RConn12 -- secondary1.16/LConn3
  Universal Bridge14/LConn1 -- secondary1.16/RConn1
  Universal Bridge15/LConn3 -- secondary1.15/RConn3
  Subsystem3/RConn10 -- secondary1.16/LConn1
  Subsystem2/RConn4 -- secondary1.21/LConn1
  Universal Bridge20/LConn1 -- secondary1.20/RConn1
  Universal Bridge19/LConn3 -- secondary1.21/RConn3
  Universal Bridge19/LConn1 -- secondary1.21/RConn1
  Subsystem2/RConn3 -- secondary1.20/LConn3
  Universal Bridge20/LConn2 -- secondary1.20/RConn2
  Subsystem2/RConn5 -- secondary1.21/LConn2
  Universal Bridge14/LConn3 -- secondary1.16/RConn3
  Subsystem2/RConn10 -- secondary1.23/LConn1
  Universal Bridge18/LConn2 -- secondary1.18/RConn2
  Subsystem3/RConn4 -- secondary1.14/LConn1
  secondary1.18/LConn1 -- Subsystem1/RConn7
  secondary1.19/LConn3 -- Subsystem1/RConn12
  Universal Bridge22/LConn3 -- secondary1.14/RConn3
  secondary1.18/LConn2 -- Subsystem1/RConn8
  Universal Bridge21/LConn3 -- secondary1.23/RConn3
  secondary1.19/LConn2 -- Subsystem1/RConn11
  Subsystem2/RConn1 -- secondary1.20/LConn1
  secondary1.19/LConn1 -- Subsystem1/RConn10
  Subsystem2/RConn6 -- secondary1.21/LConn3
  secondary1.18/LConn3 -- Subsystem1/RConn9
  Universal Bridge17/LConn1 -- secondary1.19/RConn1
  Universal Bridge19/LConn2 -- secondary1.21/RConn2
  Universal Bridge17/LConn2 -- secondary1.19/RConn2
  Subsystem3/RConn5 -- secondary1.14/LConn2
  Subsystem3/RConn3 -- secondary1.24/LConn3
  Universal Bridge18/LConn1 -- secondary1.18/RConn1
  Universal Bridge24/LConn3 -- secondary1.24/RConn3
  secondary1.13/LConn1 -- Subsystem1/RConn1
  Universal Bridge23/LConn1 -- secondary1.13/RConn1
  Universal Bridge13/LConn2 -- secondary1.17/RConn2
  Universal Bridge17/LConn3 -- secondary1.19/RConn3
  Universal Bridge23/LConn3 -- secondary1.13/RConn3
  Universal Bridge13/LConn3 -- secondary1.17/RConn3
  Universal Bridge13/LConn1 -- secondary1.17/RConn1
  Subsystem3/RConn1 -- secondary1.24/LConn1
  secondary1.13/LConn3 -- Subsystem1/RConn3
  secondary1.17/LConn1 -- Subsystem1/RConn4
  secondary1.13/LConn2 -- Subsystem1/RConn2
  secondary1.17/LConn3 -- Subsystem1/RConn6
  Universal Bridge23/LConn2 -- secondary1.13/RConn2
  Universal Bridge20/LConn3 -- secondary1.20/RConn3
  Universal Bridge18/LConn3 -- secondary1.18/RConn3
  secondary1.17/LConn2 -- Subsystem1/RConn5
  Subsystem2/RConn2 -- secondary1.20/LConn2
  Universal Bridge13/RConn2 -- IGCT17/LConn2 -- C13/RConn1
  Universal Bridge13/RConn1 -- IGCT17/LConn1 -- C13/LConn1
  Subsystem4/RConn2 -- IGCT13/LConn2 -- C22/RConn1
  C22/LConn1 -- IGCT13/LConn1 -- Subsystem4/RConn1
  Universal Bridge17/RConn2 -- IGCT19/LConn2 -- C17/RConn1
  Universal Bridge17/RConn1 -- IGCT19/LConn1 -- C17/LConn1
  Universal Bridge18/RConn2 -- IGCT18/LConn2 -- C18/RConn1
  Universal Bridge18/RConn1 -- C18/LConn1 -- IGCT18/LConn1
  C19/RConn1 -- Universal Bridge19/RConn2 -- IGCT21/LConn2
  C19/LConn1 -- Universal Bridge19/RConn1 -- IGCT21/LConn1
  C20/LConn1 -- IGCT20/LConn1 -- Universal Bridge20/RConn1
  C20/RConn1 -- IGCT20/LConn2 -- Universal Bridge20/RConn2
  Universal Bridge21/RConn2 -- IGCT23/LConn2 -- C21/RConn1
  Universal Bridge21/RConn1 -- IGCT23/LConn1 -- C21/LConn1
  Universal Bridge16/RConn2 -- IGCT22/LConn2 -- C16/RConn1
  C16/LConn1 -- Universal Bridge16/RConn1 -- IGCT22/LConn1
  Universal Bridge22/RConn2 -- IGCT14/LConn2 -- C23/RConn1
  Universal Bridge22/RConn1 -- IGCT14/LConn1 -- C23/LConn1
  C24/RConn1 -- Universal Bridge24/RConn2 -- IGCT24/LConn2
  C24/LConn1 -- IGCT24/LConn1 -- Universal Bridge24/RConn1
  C14/RConn1 -- Universal Bridge14/RConn2 -- IGCT16/LConn2
  C14/LConn1 -- Universal Bridge14/RConn1 -- IGCT16/LConn1
  C15/LConn1 -- IGCT15/LConn1 -- Universal Bridge15/RConn1
  C15/RConn1 -- IGCT15/LConn2 -- Universal Bridge15/RConn2
  IGCT16/RConn2 -- Voltage Measurement6/LConn2 -- Voltage Measurement5/LConn2 -- Voltage Measurement4/LConn2 -- Voltage Measurement7/LConn2 -- IGCT19/RConn2 -- IGCT23/RConn2
  IGCT15/RConn1 -- IGCT14/RConn2
  IGCT24/RConn2 -- IGCT14/RConn1
  IGCT23/RConn1 -- IGCT22/RConn2
  IGCT15/RConn2 -- IGCT16/RConn1
  IGCT21/RConn2 -- IGCT22/RConn1
  IGCT21/RConn1 -- IGCT20/RConn2
  IGCT18/RConn1 -- IGCT17/RConn2
  IGCT19/RConn1 -- IGCT18/RConn2
  Universal Bridge23/RConn2 -- Subsystem4/LConn2
  Universal Bridge23/RConn1 -- Subsystem4/LConn1
  IGCT17/RConn1 -- IGCT13/RConn2
  Current Measurement5/LConn1 -- Voltage Measurement6/LConn1 -- IGCT24/RConn1
  Voltage Measurement4/LConn1 -- Voltage Measurement3/LConn1 -- Current Measurement3/LConn1 -- Voltage Measurement7/LConn1 -- IGCT13/RConn1
  Voltage Measurement3/LConn2 -- Voltage Measurement5/LConn1 -- IGCT20/RConn1 -- Current Measurement4/LConn1
  Current Measurement3/RConn1 -- LOAD1/LConn1
  Current Measurement5/RConn1 -- LOAD1/LConn3
  LOAD1/LConn2 -- Current Measurement4/RConn1
  grid1/LConn3 -- 3-Phase Programmable Voltage Source7/RConn3
  grid1/LConn2 -- 3-Phase Programmable Voltage Source7/RConn2
  grid1/LConn1 -- 3-Phase Programmable Voltage Source7/RConn1
  grid1/RConn2 -- Subsystem1/LConn2 -- Subsystem3/LConn2 -- Subsystem2/LConn2
  grid1/RConn1 -- Subsystem3/LConn1 -- Subsystem1/LConn1 -- Subsystem2/LConn1
  grid1/RConn3 -- Subsystem1/LConn3 -- Subsystem3/LConn3 -- Subsystem2/LConn3

== system model_sim_CHBjt9/9 ==
  -2/3*pi : Subsystem
  0 : Subsystem
  2/3*pi : Subsystem
  Sine Wave : Sin  Amplitude=m*1000  Frequency=f*2*pi  Phase=2/3*pi  SampleTime=0
  Sine Wave1 : Sin  Amplitude=m*1000  Frequency=f*2*pi  SampleTime=0
  Sine Wave2 : Sin  Amplitude=m*1000  Frequency=f*2*pi  Phase=-2/3*pi  SampleTime=0
  Subsystem : Subsystem
  Output : Outport
  Output1 : Outport  Port=2
  Output2 : Outport  Port=3
  Output3 : Outport  Port=4
  Output4 : Outport  Port=5
  Output5 : Outport  Port=6
  Output6 : Outport  Port=7
  Output7 : Outport  Port=8
  Output8 : Outport  Port=9
  Output9 : Outport  Port=10
  Output10 : Outport  Port=11
  Output11 : Outport  Port=12
  wires:
  Subsystem/3(Out3) -> -2/3*pi/1(In1)
  Subsystem/2(Out2) -> 0/1(In1)
  Subsystem/1(Out1) -> 2/3*pi/1(In1)
  Sine Wave2/1 -> Subsystem/3(In3)
  Sine Wave1/1 -> Subsystem/2(In2)
  Sine Wave/1 -> Subsystem/1(In1)
  2/3*pi/1(Output) -> Output/1
  0/1(Out1) -> Output4/1
  -2/3*pi/1(Output8) -> Output8/1
  -2/3*pi/2(Output9) -> Output9/1
  -2/3*pi/3(Output10) -> Output10/1
  -2/3*pi/4(Output11) -> Output11/1
  0/2(Output5) -> Output5/1
  0/3(Output6) -> Output6/1
  0/4(Output7) -> Output7/1
  2/3*pi/2(Output1) -> Output1/1
  2/3*pi/3(Output2) -> Output2/1
  2/3*pi/4(Output3) -> Output3/1

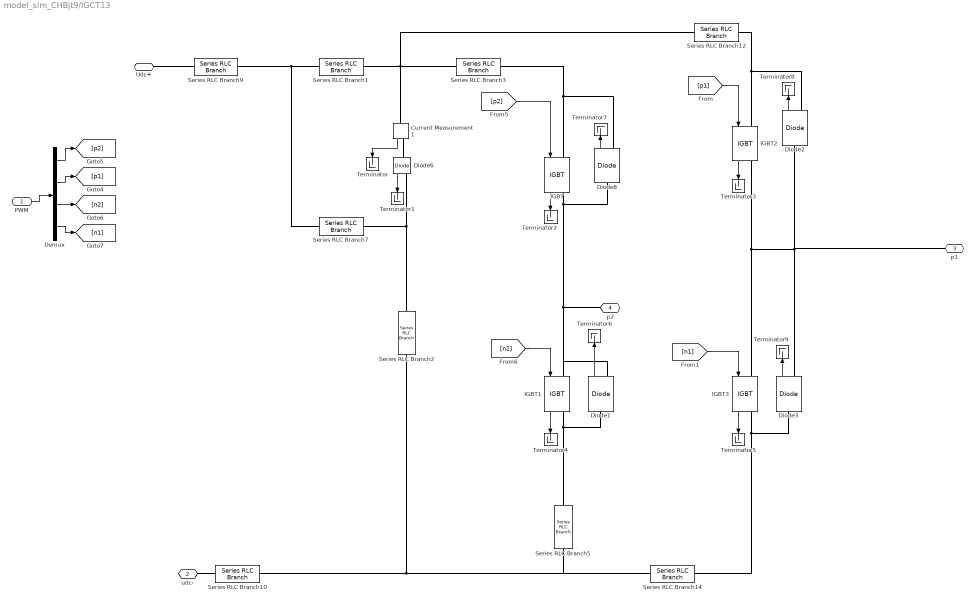
== system model_sim_CHBjt9/IGCT13 ==
  PWM : Inport
  Current Measurement1 : spsCurrentMeasurementLib/Current Measurement  PhasorSimulation=off  OutputType=Complex  PSBequivalent=0
  Demux : Demux
  Diode{1..3,6,8} (5 alike) : spsDiodeLib/Diode  Ron=rto  Lon=0  Vf=vto  IC=0  UseSnubber=off  Rs=500  Cs=250e-9  Measurements=on
  IGBT{,1..3} (4 alike) : spsIGBTLib/IGBT  Ron=rt  Lon=0  Vf=vt  Tf=1e-6  Tt=2e-6  IC=0  Rs=1e5  Cs=inf  Measurements=on
  Series RLC Branch1 : spsSeriesRLCBranchLib/Series RLC Branch  LConnTagsString=__new0  RConnTagsString=__new0  BranchType=RL  Resistance=1e-5  Inductance=3.0E-6  SetiL0=off  InitialCurrent=0  Capacitance=1e-6  Setx0=off  InitialVoltage=0  Measurements=None
  Series RLC Branch10 : spsSeriesRLCBranchLib/Series RLC Branch  LConnTagsString=__new0  RConnTagsString=__new0  BranchType=L  Resistance=1  Inductance=0.4e-6  SetiL0=off  InitialCurrent=0  Capacitance=1e-6  Setx0=off  InitialVoltage=0  Measurements=None
  Series RLC Branch12 : spsSeriesRLCBranchLib/Series RLC Branch  LConnTagsString=__new0  RConnTagsString=__new0  BranchType=RL  Resistance=1e-5  Inductance=1E-9  SetiL0=off  InitialCurrent=0  Capacitance=1e-6  Setx0=off  InitialVoltage=0  Measurements=None
  Series RLC Branch14 : spsSeriesRLCBranchLib/Series RLC Branch  LConnTagsString=__new0  RConnTagsString=__new0  BranchType=L  Resistance=1  Inductance=1E-7  SetiL0=off  InitialCurrent=0  Capacitance=1e-6  Setx0=off  InitialVoltage=0  Measurements=None
  Series RLC Branch2 : spsSeriesRLCBranchLib/Series RLC Branch  LConnTagsString=__new0  RConnTagsString=__new0  BranchType=RC  Resistance=1e-5  Inductance=20e-6  SetiL0=off  InitialCurrent=0  Capacitance=17e-6  Setx0=off  InitialVoltage=0  Measurements=None
  Series RLC Branch3 : spsSeriesRLCBranchLib/Series RLC Branch  LConnTagsString=__new0  RConnTagsString=__new0  BranchType=RL  Resistance=1e-5  Inductance=1E-9  SetiL0=off  InitialCurrent=0  Capacitance=1e-6  Setx0=off  InitialVoltage=0  Measurements=None
  Series RLC Branch5 : spsSeriesRLCBranchLib/Series RLC Branch  LConnTagsString=__new0  RConnTagsString=__new0  BranchType=L  Resistance=1  Inductance=1E-7  SetiL0=off  InitialCurrent=0  Capacitance=1e-6  Setx0=off  InitialVoltage=0  Measurements=None
  Series RLC Branch7 : spsSeriesRLCBranchLib/Series RLC Branch  LConnTagsString=__new0  RConnTagsString=__new0  BranchType=RL  Resistance=0.6  Inductance=1e-6  SetiL0=off  InitialCurrent=0  Capacitance=1e-6  Setx0=off  InitialVoltage=0  Measurements=None
  Series RLC Branch9 : spsSeriesRLCBranchLib/Series RLC Branch  LConnTagsString=__new0  RConnTagsString=__new0  BranchType=L  Resistance=1  Inductance=0.4e-6  SetiL0=off  InitialCurrent=0  Capacitance=1e-6  Setx0=off  InitialVoltage=0  Measurements=None
  Terminator{,1..9} (10 alike) : Terminator
  Udc+ : PMIOPort  Side=Left
  udc- : PMIOPort  Port=2  Side=Left
  p1 : PMIOPort  Port=3  Side=Right
  p2 : PMIOPort  Port=4  Side=Right
  wires:
  Demux/4 -> [n1]
  Demux/2 -> [p1]
  Demux/1 -> [p2]
  PWM/1 -> Demux/1
  Demux/3 -> [n2]
  Diode6/1 -> Terminator1/1
  Diode1/1 -> Terminator6/1
  Diode8/1 -> Terminator7/1
  [p2] -> IGBT/1
  Diode2/1 -> Terminator8/1
  Current Measurement1/1 -> Terminator/1
  [p1] -> IGBT2/1
  [n2] -> IGBT1/1
  IGBT/1 -> Terminator2/1
  IGBT2/1 -> Terminator3/1
  IGBT1/1 -> Terminator4/1
  [n1] -> IGBT3/1
  IGBT3/1 -> Terminator5/1
  Diode3/1 -> Terminator9/1
  connections:
  IGBT/RConn1 -- Diode8/LConn1 -- Diode1/RConn1 -- IGBT1/LConn1 -- p2/RConn1
  Series RLC Branch9/RConn1 -- Series RLC Branch7/LConn1 -- Series RLC Branch1/LConn1
  Series RLC Branch2/RConn1 -- Series RLC Branch10/RConn1 -- Series RLC Branch14/LConn1 -- Series RLC Branch5/LConn1
  IGBT2/RConn1 -- IGBT3/LConn1 -- Diode3/RConn1 -- Diode2/LConn1 -- p1/RConn1
  IGBT2/LConn1 -- Series RLC Branch12/RConn1 -- Diode2/RConn1
  Current Measurement1/RConn1 -- Diode6/LConn1
  IGBT1/RConn1 -- Series RLC Branch5/RConn1 -- Diode1/LConn1
  Diode8/RConn1 -- IGBT/LConn1 -- Series RLC Branch3/RConn1
  Series RLC Branch14/RConn1 -- IGBT3/RConn1 -- Diode3/LConn1
  Series RLC Branch12/LConn1 -- Series RLC Branch3/LConn1 -- Series RLC Branch1/RConn1 -- Current Measurement1/LConn1
  Series RLC Branch2/LConn1 -- Series RLC Branch7/RConn1 -- Diode6/RConn1
  Series RLC Branch9/LConn1 -- Udc+/RConn1
  Series RLC Branch10/LConn1 -- udc-/RConn1

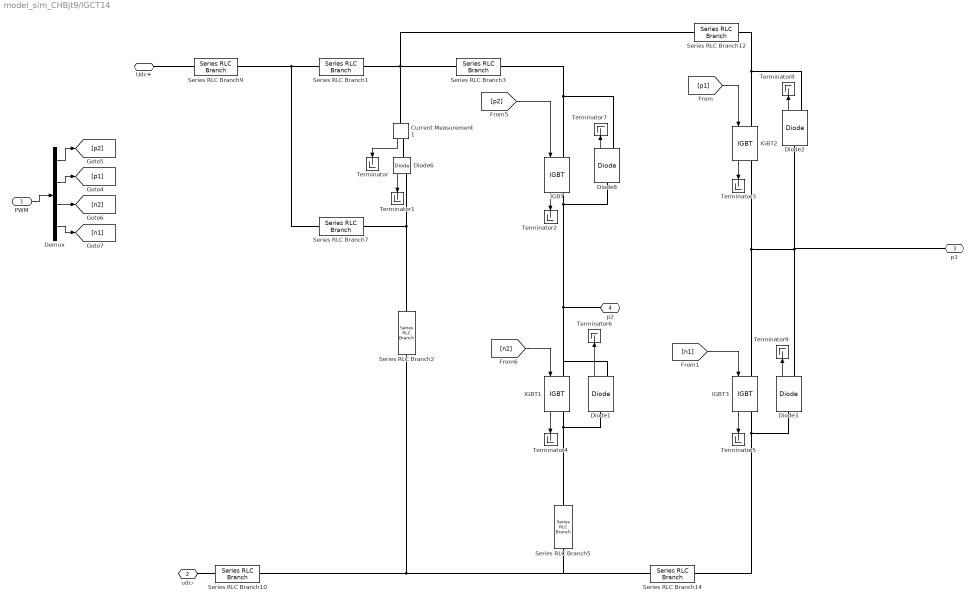
== system model_sim_CHBjt9/IGCT14 ==
  PWM : Inport
  Current Measurement1 : spsCurrentMeasurementLib/Current Measurement  PhasorSimulation=off  OutputType=Complex  PSBequivalent=0
  Demux : Demux
  Diode{1..3,6,8} (5 alike) : spsDiodeLib/Diode  Ron=rto  Lon=0  Vf=vto  IC=0  UseSnubber=off  Rs=500  Cs=250e-9  Measurements=on
  IGBT{,1..3} (4 alike) : spsIGBTLib/IGBT  Ron=rt  Lon=0  Vf=vt  Tf=1e-6  Tt=2e-6  IC=0  Rs=1e5  Cs=inf  Measurements=on
  Series RLC Branch1 : spsSeriesRLCBranchLib/Series RLC Branch  LConnTagsString=__new0  RConnTagsString=__new0  BranchType=RL  Resistance=1e-5  Inductance=3.0E-6  SetiL0=off  InitialCurrent=0  Capacitance=1e-6  Setx0=off  InitialVoltage=0  Measurements=None
  Series RLC Branch10 : spsSeriesRLCBranchLib/Series RLC Branch  LConnTagsString=__new0  RConnTagsString=__new0  BranchType=L  Resistance=1  Inductance=0.4e-6  SetiL0=off  InitialCurrent=0  Capacitance=1e-6  Setx0=off  InitialVoltage=0  Measurements=None
  Series RLC Branch12 : spsSeriesRLCBranchLib/Series RLC Branch  LConnTagsString=__new0  RConnTagsString=__new0  BranchType=RL  Resistance=1e-5  Inductance=1E-9  SetiL0=off  InitialCurrent=0  Capacitance=1e-6  Setx0=off  InitialVoltage=0  Measurements=None
  Series RLC Branch14 : spsSeriesRLCBranchLib/Series RLC Branch  LConnTagsString=__new0  RConnTagsString=__new0  BranchType=L  Resistance=1  Inductance=1E-7  SetiL0=off  InitialCurrent=0  Capacitance=1e-6  Setx0=off  InitialVoltage=0  Measurements=None
  Series RLC Branch2 : spsSeriesRLCBranchLib/Series RLC Branch  LConnTagsString=__new0  RConnTagsString=__new0  BranchType=RC  Resistance=1e-5  Inductance=20e-6  SetiL0=off  InitialCurrent=0  Capacitance=17e-6  Setx0=off  InitialVoltage=0  Measurements=None
  Series RLC Branch3 : spsSeriesRLCBranchLib/Series RLC Branch  LConnTagsString=__new0  RConnTagsString=__new0  BranchType=RL  Resistance=1e-5  Inductance=1E-9  SetiL0=off  InitialCurrent=0  Capacitance=1e-6  Setx0=off  InitialVoltage=0  Measurements=None
  Series RLC Branch5 : spsSeriesRLCBranchLib/Series RLC Branch  LConnTagsString=__new0  RConnTagsString=__new0  BranchType=L  Resistance=1  Inductance=1E-7  SetiL0=off  InitialCurrent=0  Capacitance=1e-6  Setx0=off  InitialVoltage=0  Measurements=None
  Series RLC Branch7 : spsSeriesRLCBranchLib/Series RLC Branch  LConnTagsString=__new0  RConnTagsString=__new0  BranchType=RL  Resistance=0.6  Inductance=1e-6  SetiL0=off  InitialCurrent=0  Capacitance=1e-6  Setx0=off  InitialVoltage=0  Measurements=None
  Series RLC Branch9 : spsSeriesRLCBranchLib/Series RLC Branch  LConnTagsString=__new0  RConnTagsString=__new0  BranchType=L  Resistance=1  Inductance=0.4e-6  SetiL0=off  InitialCurrent=0  Capacitance=1e-6  Setx0=off  InitialVoltage=0  Measurements=None
  Terminator{,1..9} (10 alike) : Terminator
  Udc+ : PMIOPort  Side=Left
  udc- : PMIOPort  Port=2  Side=Left
  p1 : PMIOPort  Port=3  Side=Right
  p2 : PMIOPort  Port=4  Side=Right
  wires:
  Demux/4 -> [n1]
  Demux/2 -> [p1]
  Demux/1 -> [p2]
  PWM/1 -> Demux/1
  Demux/3 -> [n2]
  Diode6/1 -> Terminator1/1
  Diode1/1 -> Terminator6/1
  Diode8/1 -> Terminator7/1
  [p2] -> IGBT/1
  Diode2/1 -> Terminator8/1
  Current Measurement1/1 -> Terminator/1
  [p1] -> IGBT2/1
  [n2] -> IGBT1/1
  IGBT/1 -> Terminator2/1
  IGBT2/1 -> Terminator3/1
  IGBT1/1 -> Terminator4/1
  [n1] -> IGBT3/1
  IGBT3/1 -> Terminator5/1
  Diode3/1 -> Terminator9/1
  connections:
  IGBT/RConn1 -- Diode8/LConn1 -- Diode1/RConn1 -- IGBT1/LConn1 -- p2/RConn1
  Series RLC Branch9/RConn1 -- Series RLC Branch7/LConn1 -- Series RLC Branch1/LConn1
  Series RLC Branch2/RConn1 -- Series RLC Branch10/RConn1 -- Series RLC Branch14/LConn1 -- Series RLC Branch5/LConn1
  IGBT2/RConn1 -- IGBT3/LConn1 -- Diode3/RConn1 -- Diode2/LConn1 -- p1/RConn1
  IGBT2/LConn1 -- Series RLC Branch12/RConn1 -- Diode2/RConn1
  Current Measurement1/RConn1 -- Diode6/LConn1
  IGBT1/RConn1 -- Series RLC Branch5/RConn1 -- Diode1/LConn1
  Diode8/RConn1 -- IGBT/LConn1 -- Series RLC Branch3/RConn1
  Series RLC Branch14/RConn1 -- IGBT3/RConn1 -- Diode3/LConn1
  Series RLC Branch12/LConn1 -- Series RLC Branch3/LConn1 -- Series RLC Branch1/RConn1 -- Current Measurement1/LConn1
  Series RLC Branch2/LConn1 -- Series RLC Branch7/RConn1 -- Diode6/RConn1
  Series RLC Branch9/LConn1 -- Udc+/RConn1
  Series RLC Branch10/LConn1 -- udc-/RConn1

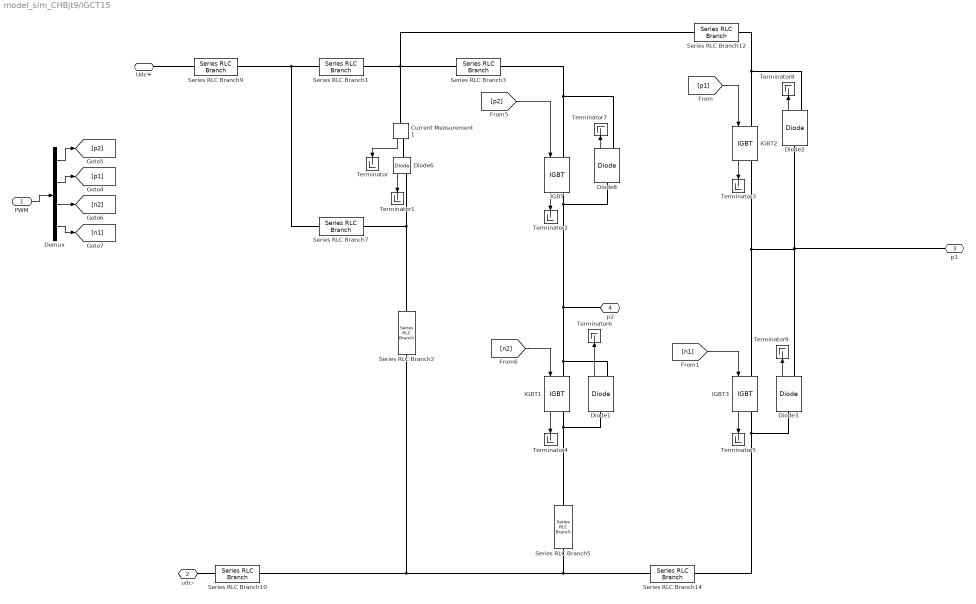
== system model_sim_CHBjt9/IGCT15 ==
  PWM : Inport
  Current Measurement1 : spsCurrentMeasurementLib/Current Measurement  PhasorSimulation=off  OutputType=Complex  PSBequivalent=0
  Demux : Demux
  Diode{1..3,6,8} (5 alike) : spsDiodeLib/Diode  Ron=rto  Lon=0  Vf=vto  IC=0  UseSnubber=off  Rs=500  Cs=250e-9  Measurements=on
  IGBT{,1..3} (4 alike) : spsIGBTLib/IGBT  Ron=rt  Lon=0  Vf=vt  Tf=1e-6  Tt=2e-6  IC=0  Rs=1e5  Cs=inf  Measurements=on
  Series RLC Branch1 : spsSeriesRLCBranchLib/Series RLC Branch  LConnTagsString=__new0  RConnTagsString=__new0  BranchType=RL  Resistance=1e-5  Inductance=3.0E-6  SetiL0=off  InitialCurrent=0  Capacitance=1e-6  Setx0=off  InitialVoltage=0  Measurements=None
  Series RLC Branch10 : spsSeriesRLCBranchLib/Series RLC Branch  LConnTagsString=__new0  RConnTagsString=__new0  BranchType=L  Resistance=1  Inductance=0.4e-6  SetiL0=off  InitialCurrent=0  Capacitance=1e-6  Setx0=off  InitialVoltage=0  Measurements=None
  Series RLC Branch12 : spsSeriesRLCBranchLib/Series RLC Branch  LConnTagsString=__new0  RConnTagsString=__new0  BranchType=RL  Resistance=1e-5  Inductance=1E-9  SetiL0=off  InitialCurrent=0  Capacitance=1e-6  Setx0=off  InitialVoltage=0  Measurements=None
  Series RLC Branch14 : spsSeriesRLCBranchLib/Series RLC Branch  LConnTagsString=__new0  RConnTagsString=__new0  BranchType=L  Resistance=1  Inductance=1E-7  SetiL0=off  InitialCurrent=0  Capacitance=1e-6  Setx0=off  InitialVoltage=0  Measurements=None
  Series RLC Branch2 : spsSeriesRLCBranchLib/Series RLC Branch  LConnTagsString=__new0  RConnTagsString=__new0  BranchType=RC  Resistance=1e-5  Inductance=20e-6  SetiL0=off  InitialCurrent=0  Capacitance=17e-6  Setx0=off  InitialVoltage=0  Measurements=None
  Series RLC Branch3 : spsSeriesRLCBranchLib/Series RLC Branch  LConnTagsString=__new0  RConnTagsString=__new0  BranchType=RL  Resistance=1e-5  Inductance=1E-9  SetiL0=off  InitialCurrent=0  Capacitance=1e-6  Setx0=off  InitialVoltage=0  Measurements=None
  Series RLC Branch5 : spsSeriesRLCBranchLib/Series RLC Branch  LConnTagsString=__new0  RConnTagsString=__new0  BranchType=L  Resistance=1  Inductance=1E-7  SetiL0=off  InitialCurrent=0  Capacitance=1e-6  Setx0=off  InitialVoltage=0  Measurements=None
  Series RLC Branch7 : spsSeriesRLCBranchLib/Series RLC Branch  LConnTagsString=__new0  RConnTagsString=__new0  BranchType=RL  Resistance=0.6  Inductance=1e-6  SetiL0=off  InitialCurrent=0  Capacitance=1e-6  Setx0=off  InitialVoltage=0  Measurements=None
  Series RLC Branch9 : spsSeriesRLCBranchLib/Series RLC Branch  LConnTagsString=__new0  RConnTagsString=__new0  BranchType=L  Resistance=1  Inductance=0.4e-6  SetiL0=off  InitialCurrent=0  Capacitance=1e-6  Setx0=off  InitialVoltage=0  Measurements=None
  Terminator{,1..9} (10 alike) : Terminator
  Udc+ : PMIOPort  Side=Left
  udc- : PMIOPort  Port=2  Side=Left
  p1 : PMIOPort  Port=3  Side=Right
  p2 : PMIOPort  Port=4  Side=Right
  wires:
  Diode3/1 -> Terminator9/1
  IGBT3/1 -> Terminator5/1
  [n1] -> IGBT3/1
  IGBT1/1 -> Terminator4/1
  IGBT2/1 -> Terminator3/1
  IGBT/1 -> Terminator2/1
  [n2] -> IGBT1/1
  [p1] -> IGBT2/1
  Current Measurement1/1 -> Terminator/1
  Diode2/1 -> Terminator8/1
  [p2] -> IGBT/1
  Diode8/1 -> Terminator7/1
  Diode1/1 -> Terminator6/1
  Diode6/1 -> Terminator1/1
  Demux/3 -> [n2]
  PWM/1 -> Demux/1
  Demux/1 -> [p2]
  Demux/2 -> [p1]
  Demux/4 -> [n1]
  connections:
  Series RLC Branch10/LConn1 -- udc-/RConn1
  Series RLC Branch9/LConn1 -- Udc+/RConn1
  Diode6/RConn1 -- Series RLC Branch7/RConn1 -- Series RLC Branch2/LConn1
  Current Measurement1/LConn1 -- Series RLC Branch1/RConn1 -- Series RLC Branch3/LConn1 -- Series RLC Branch12/LConn1
  Diode3/LConn1 -- IGBT3/RConn1 -- Series RLC Branch14/RConn1
  Series RLC Branch3/RConn1 -- IGBT/LConn1 -- Diode8/RConn1
  Diode1/LConn1 -- Series RLC Branch5/RConn1 -- IGBT1/RConn1
  Current Measurement1/RConn1 -- Diode6/LConn1
  Diode2/RConn1 -- Series RLC Branch12/RConn1 -- IGBT2/LConn1
  p1/RConn1 -- Diode2/LConn1 -- Diode3/RConn1 -- IGBT3/LConn1 -- IGBT2/RConn1
  Series RLC Branch5/LConn1 -- Series RLC Branch14/LConn1 -- Series RLC Branch10/RConn1 -- Series RLC Branch2/RConn1
  Series RLC Branch1/LConn1 -- Series RLC Branch7/LConn1 -- Series RLC Branch9/RConn1
  p2/RConn1 -- IGBT1/LConn1 -- Diode1/RConn1 -- Diode8/LConn1 -- IGBT/RConn1
